simulink model "basic_control_system"  (R2024a)
settings: Solver=VariableStepAuto  StartTime=0.0  StopTime=10.0  RelTol=1e-3
undefined symbols (not defined in the file or in its folder): K, kd, ks, m, N, Td, Ti
settings Model: Creator=saran  LastModifiedBy=saran

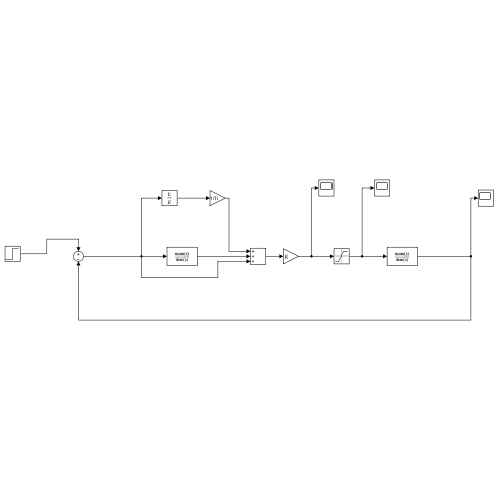
[thumbnail: Simulink's stored preview of the top-level diagram]
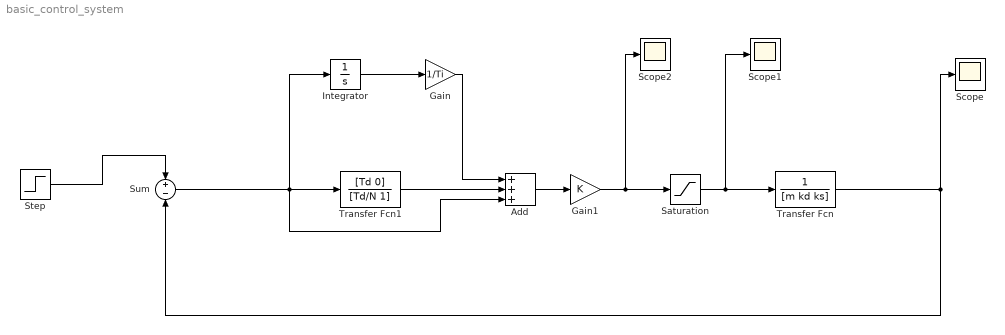
== system basic_control_system ==
  Add : Sum  Inputs=+++
  Gain : Gain  Gain=1/Ti
  Gain1 : Gain  Gain=K
  Integrator : Integrator
  Saturation : Saturate  UpperLimit=50  LowerLimit=-50
  Scope : Scope
  Scope1 : Scope
  Scope2 : Scope
  Step : Step  SampleTime=0
  Sum : Sum  Inputs=+-
  Transfer Fcn : TransferFcn  Denominator=[m kd ks]
  Transfer Fcn1 : TransferFcn  Numerator=[Td 0]  Denominator=[Td/N 1]
  wires:
  Transfer Fcn/1 -> Sum/2, Scope/1
  Step/1 -> Sum/1
  Sum/1 -> Add/3, Transfer Fcn1/1, Integrator/1
  Integrator/1 -> Gain/1
  Add/1 -> Gain1/1
  Transfer Fcn1/1 -> Add/2
  Gain/1 -> Add/1
  Gain1/1 -> Scope2/1, Saturation/1
  Saturation/1 -> Scope1/1, Transfer Fcn/1
